simulink model "mrs_ptfsc_mdl"  (Simulink 8.3)
settings: Solver=ode45  StartTime=0.0  StopTime=10  RelTol=1e-3
settings Model: Creator=Administrator  LastModifiedBy=JimmyChen
settings DataIOCC: SignalLoggingSaveFormat=Dataset
settings DebuggingCC: UnderspecifiedInitializationDetection=Simplified  StateNameClashWarn=none
settings GRTTargetCC: CombineOutputUpdateFcns=on  GRTInterface=off

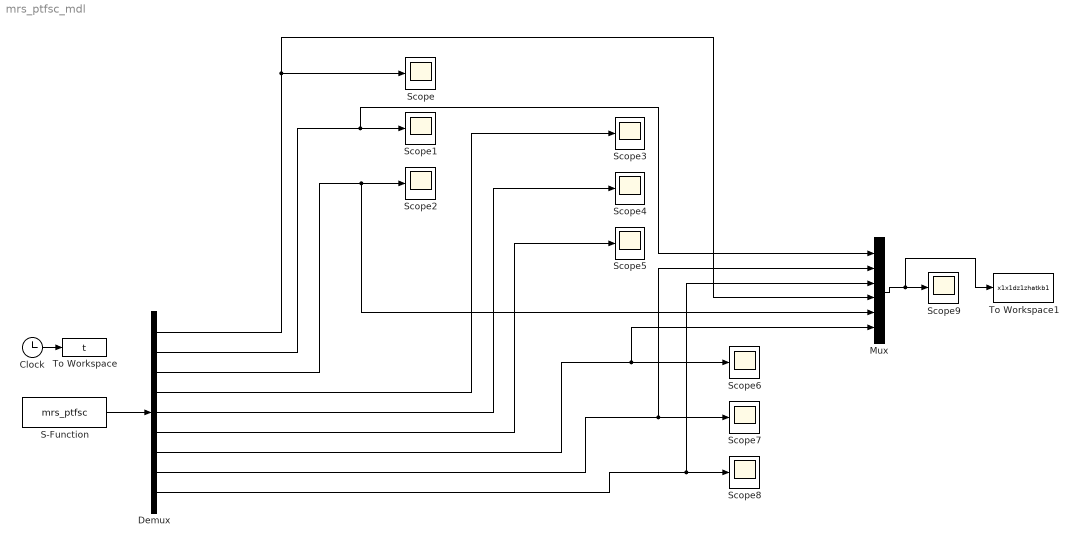
== system mrs_ptfsc_mdl ==
  Clock : Clock
  Demux : Demux  Outputs=9
  Mux : Mux  Inputs=6
  S-Function : S-Function  FunctionName=mrs_ptfsc  EnableBusSupport=off
  Scope{,1..9} (10 alike) : Scope
      Scope2 settings: SaveName=ScopeData2
      Scope3 settings: SaveName=ScopeData3
      Scope4 settings: SaveName=ScopeData4
      Scope5 settings: SaveName=ScopeData5
      Scope6 settings: SaveName=ScopeData6
      Scope7 settings: SaveName=ScopeData7
      Scope8 settings: SaveName=ScopeData8
      Scope9 settings: SaveName=ScopeData9
  To Workspace : ToWorkspace  VariableName=t  SaveFormat=Timeseries  SampleTime=-1
  To Workspace1 : ToWorkspace  VariableName=x1x1dz1zhatkb1  SaveFormat=Timeseries  SampleTime=-1
  wires:
  S-Function/1 -> Demux/1
  Clock/1 -> To Workspace/1
  Demux/1 -> Scope/1, Mux/4
  Demux/2 -> Mux/1, Scope1/1
  Demux/3 -> Mux/5, Scope2/1
  Demux/4 -> Scope3/1
  Demux/5 -> Scope4/1
  Demux/6 -> Scope5/1
  Demux/7 -> Mux/6, Scope6/1
  Demux/8 -> Mux/2, Scope7/1
  Demux/9 -> Scope8/1, Mux/3
  Mux/1 -> To Workspace1/1, Scope9/1
